simulink model "Ex5_3_iii_iv"  (R2022b)
settings: Solver=ode4  StartTime=0.0  StopTime=10.0  FixedStep=0.001  RelTol=1e-3
undefined symbols (not defined in the file or in its folder): par
settings Model: Creator=super  LastModifiedBy=15043
settings ModelReferenceCC: EnableRefExpFcnMdlSchedulingChecks=on

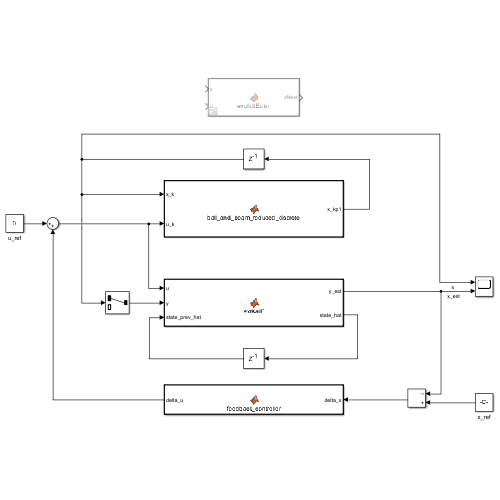
[thumbnail: Simulink's stored preview of the top-level diagram]
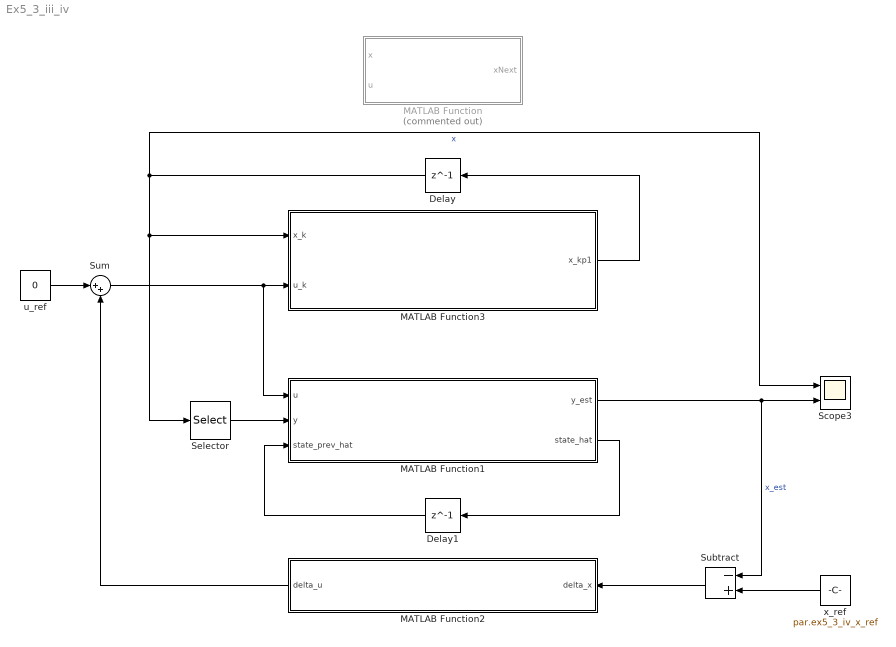
== system Ex5_3_iii_iv ==
  Delay : Delay  DelayLength=1  InitialCondition=par.ex5_3_iii_x0
  Delay1 : Delay  DelayLength=1  InitialCondition=par.ex5_3_iii_x0_hat  UseCircularBuffer=on
  MATLAB Function : MATLAB Function  Commented=on  TreatAsAtomicUnit=on
  MATLAB Function1 : MATLAB Function  TreatAsAtomicUnit=on
  MATLAB Function2 : MATLAB Function  TreatAsAtomicUnit=on
  MATLAB Function3 : MATLAB Function  TreatAsAtomicUnit=on
  Scope3 : Scope  NumInputPorts=2
  Selector : Selector  InputPortWidth=2  IndexOptions=Index vector (dialog)  Indices=[1]  OutputSizes=1
  Subtract : Sum  Inputs=-+
  Sum : Sum  Inputs=|++
  u_ref : Constant  Value=0
  x_ref : Constant  Value=par.ex5_3_iv_x_ref
  wires:
  Delay/1 -> MATLAB Function3/1(x_k), Selector/1, Scope3/1  "x"
  MATLAB Function1/2(state_hat) -> Delay1/1
  Delay1/1 -> MATLAB Function1/3(state_prev_hat)
  Selector/1 -> MATLAB Function1/2(y)
  MATLAB Function1/1(y_est) -> Subtract/1, Scope3/2  "x_est"
  Subtract/1 -> MATLAB Function2/1(delta_x)
  u_ref/1 -> Sum/1
  Sum/1 -> MATLAB Function1/1(u), MATLAB Function3/2(u_k)
  MATLAB Function3/1(x_kp1) -> Delay/1
  MATLAB Function2/1(delta_u) -> Sum/2
  x_ref/1 -> Subtract/2

== matlab function Ex5_3_iii_iv/MATLAB Function2 ==
  data: delta_x input; delta_u output; par parameter
function delta_u = feedback_controller(delta_x,par)

k = par.ex5_3_iv_k;
delta_u = k*delta_x;

end

== matlab function Ex5_3_iii_iv/MATLAB Function ==
  data: x input; u input; xNext output; par parameter
function xNext = explicitEuler(x,u,par)
 
    h = par.timeStep;
    xNext = x + h*reducedModel( x, u, par);

end

function dx = reducedModel( x, u, par )
    
    % system parameters   
    g = par.g;

    % States vector
    x2 = x(2);

    % Preallocate
    dx = zeros(2,1);

    % reduced model
    dx(1) = x2;
    dx(2) = -(5/7)*g*sin(u);
end

== matlab function Ex5_3_iii_iv/MATLAB Function1 ==
  data: y_est output; u input; state_hat output; y input; state_prev_hat input; par parameter
function [y_est, state_hat] = extKalF(u, y, state_prev_hat, par )
    
    R = par.R;          % Measurement covariance matrix
    Q = par.Q;          % Process covariance matrix

    ts = par.timeStep;  % discretization timestep for the explicit euler

    h = @(x) [x(1)];    % As we only measure the first state
    
    H = [1 0];          % Measurement Jacobian        
    dF = [ 0 1; 0 0];   % State jacobian    
    
    x_hat_prev = state_prev_hat(1:2, :);
    P_prev = reshape( state_prev_hat(3:end), 2,2);
    
    % discretize the nonlinear model
    fd = x_hat_prev + ts*f( x_hat_prev, u, par );
    
    % discretize the jacobian
    F = eye(2) + ts*dF;

    %%%%%% Predict step %%%%%%
    x_hatm = fd;
    Pm = F*P_prev*F' + Q;
    
    %%%%%% Update step %%%%%%
    K = Pm*H'/((H*Pm*H'+ R));         % Kalman gain
    
    x_hat = x_hatm + K*(y-h(x_hatm));   
    P = ( eye(2) - K*H)*Pm ;
         
    state_hat = [x_hat; P(:);];
    y_est = x_hat_prev;
 end


function dx = f( x, u, par )
    
    % system parameters   
    g = par.g;

    % States vector
    x2 = x(2);

    % Preallocate
    dx = zeros(2,1);

    % reduced model
    dx(1) = x2;
    dx(2) = -(5/7)*g*sin(u);
end

== matlab function Ex5_3_iii_iv/MATLAB Function3 ==
  data: x_k input; u_k input; x_kp1 output; par parameter
function x_kp1 = ball_and_beam_reduced_discrete(x_k, u_k, par)
%#codegen
x_kp1 = ball_and_beam_reduced_discrete(x_k, u_k, par);
